simulink model "AM_07_model_pretvornik_FOC"  (R2016a)
settings: Solver=ode23  StartTime=0.0  StopTime=1  FixedStep=25e-9  MaxStep=1/(20*Fstikalna)  RelTol=1e-2
InitFcn:
  | parametriAM
values from neighbouring files (symbols this model uses):
  Imrn = 7.4    [parametriAM.m]
  In = 12.7    [parametriAM.m]
  Ismax = In*sqrt(2)    [parametriAM.m]
  J = 0.019    [parametriAM.m]    (also in podatki.m = 0.01)
  Ki_tok = 5.0    (= 5)    [parametriAM.m]
  Ki_wr = 1000    [parametriAM.m]
  Kp_tok = 0.05    [parametriAM.m]
  Kp_wr = 50    [parametriAM.m]
  Lm = 0.0493    [parametriAM.m]    (also in podatki.m = 0.2342)
  Lr = 0.05315    [parametriAM.m]    (also in podatki.m = 0.2449)
  Ls = 0.05315    [parametriAM.m]    (also in podatki.m = 0.2449)
  Lst = sigma*Ls    (= 0.00742111947319)    [parametriAM.m]
  pp = 3    [parametriAM.m]    (also in podatki.m = 2)
  sigma = 1 - 1/((1+sigmaR)*(1+sigmaS))    (= 0.13962595434)    [parametriAM.m]
  Tr = Lr/Rr    (= 0.0771407837446)    [parametriAM.m]
  Tstikalna = 1/Fstikalna    (= 0.0001)    [parametriAM.m]
  Udc = Un*sqrt(2/3*2)    [parametriAM.m]
  Un = 216    [parametriAM.m]
  wb_upper_limit_field_weaking = sqrt((Ls^2+Lst^2)/(2*Lst^2*Ls^2))*Un/Ismax    [parametriAM.m]
  wn = Udc/sqrt(Ls^2*(Imrn)^2+Lst^2*(Ismax^2-(Imrn)^2))    [maximalnaelipsa.m]    (also in parametriAM.m = Udc/sqrt(Ls^2*(Imrn)^2+Lst^2*(Ismax^2-(Imrn)^2))/pp/sqrt(2))
undefined symbols (not defined in the file or in its folder): DiscIntNeverNeededParam
undefined symbols (not defined in the file): Rr, Rs
libraries: simulink x23, simulink_extras x3
(part 2 of 2)

== system AM_07_model_pretvornik_FOC/Regulacija1/tokovni_model ==
  I_123 : Inport
  wr : Inport  Port=2
  Clarke : Subsystem
  Demux : Demux  Outputs=2
  Discrete-Time Integrator : DiscreteIntegrator  SampleTime=-1  ICPrevOutput=DiscIntNeverNeededParam  ICPrevScaledInput=DiscIntNeverNeededParam
  Gain : Gain  Gain=pp
  Park : Subsystem
  Terminator : Terminator
  eq 5.39 : Subsystem
  eq 5.40 : Subsystem
  I_dq : Outport
  Imr : Outport  Port=2
  ro : Outport  Port=3
  wires:
  wr/1 -> Gain/1
  eq 5.39/2(dImr/dt) -> Terminator/1
  Discrete-Time Integrator/1 -> Park/2(kot), ro/1
  eq 5.40/1(wmr) -> Discrete-Time Integrator/1
  Gain/1 -> eq 5.40/3(wr_el)
  Demux/2 -> eq 5.40/2(Isq)
  eq 5.39/1(Imr) -> Imr/1, eq 5.40/1(Imr)
  Demux/1 -> eq 5.39/1(Isd)
  I_123/1 -> Clarke/1(U_123)
  Clarke/1(U_ab) -> Park/1(U_ab)
  Park/1(U_dq) -> Demux/1, I_dq/1

== system AM_07_model_pretvornik_FOC/Regulacija2/Inverzni Park ==
  U_dq : Inport
  kot : Inport  Port=2
  Demux : Demux  Outputs=2
  Mux : Mux  Inputs=2
  "Sum1 " : Sum  Inputs=+-  SaturateOnIntegerOverflow=on  InputSameDT=on  OutDataTypeStr=Inherit: Same as first input
  Sum2 : Sum  SaturateOnIntegerOverflow=on  InputSameDT=on  OutDataTypeStr=Inherit: Same as first input
  cos : Fcn  Expr=cos(u)
  sin : Fcn  Expr=sin(u)
  x_d*cos : Product  SaturateOnIntegerOverflow=on  RndMeth=Zero  InputSameDT=on  OutDataTypeStr=Inherit: Same as first input
  x_d*sin : Product  SaturateOnIntegerOverflow=on  RndMeth=Zero  InputSameDT=on  OutDataTypeStr=Inherit: Same as first input
  x_q*cos : Product  SaturateOnIntegerOverflow=on  RndMeth=Zero  InputSameDT=on  OutDataTypeStr=Inherit: Same as first input
  "x_q*sin " : Product  SaturateOnIntegerOverflow=on  RndMeth=Zero  InputSameDT=on  OutDataTypeStr=Inherit: Same as first input
  U_ab : Outport
  wires:
  kot/1 -> sin/1, cos/1
  Sum2/1 -> Mux/2
  "Sum1 "/1 -> Mux/1
  x_d*sin/1 -> Sum2/1
  x_q*cos/1 -> Sum2/2
  "x_q*sin "/1 -> "Sum1 "/2
  x_d*cos/1 -> "Sum1 "/1
  sin/1 -> x_d*sin/2, "x_q*sin "/2
  cos/1 -> x_d*cos/2, x_q*cos/2
  Demux/2 -> x_q*cos/1, "x_q*sin "/1
  Demux/1 -> x_d*cos/1, x_d*sin/1
  U_dq/1 -> Demux/1
  Mux/1 -> U_ab/1

== system AM_07_model_pretvornik_FOC/Regulacija2/TechniqueA2 ==
  wmr : Inport
  Abs : Abs
  Add : Sum
  Constant : Constant  Value=wn
  Constant1 : Constant  Value=0.000001
  Constant2 : Constant  Value=Imrn
  Divide : Product  Inputs=*/
  Product : Product
  Saturation : Saturate  UpperLimit=+Imrn*sqrt(2)  LowerLimit=-Imrn*sqrt(2)
  Saturation2 : Saturate  UpperLimit=wb_upper_limit_field_weaking  LowerLimit=-wb_upper_limit_field_weaking
  Nemec : Outport
  wires:
  Saturation2/1 -> Abs/1
  Saturation/1 -> Nemec/1
  Constant1/1 -> Add/2
  Abs/1 -> Add/1
  Add/1 -> Divide/2
  Constant/1 -> Divide/1
  Product/1 -> Saturation/1
  Divide/1 -> Product/2
  Constant2/1 -> Product/1
  wmr/1 -> Saturation2/1

== system AM_07_model_pretvornik_FOC/Regulacija2/hitrostna regulacija ==
  ref : Inport
  fdb : Inport  Port=2
  1/Ti : Gain  Gain=Ki_wr  SaturateOnIntegerOverflow=on  OutDataTypeStr=Inherit: Same as input  ParamDataTypeStr=Inherit: Same as input
  Abs : Abs
  Add2 : Sum  Inputs=+-
  Compare To Zero : simulink/Logic and Bit Operations/Compare To Zero  relop=<=  OutDataTypeStr=boolean
  Discrete-Time Integrator : DiscreteIntegrator  SampleTime=-1  ICPrevOutput=DiscIntNeverNeededParam  ICPrevScaledInput=DiscIntNeverNeededParam
  Kp : Gain  Gain=Kp_wr  SaturateOnIntegerOverflow=on  OutDataTypeStr=Inherit: Same as input  ParamDataTypeStr=Inherit: Same as input
  Product : Product
  Saturation : Saturate  UpperLimit=+sqrt((In^2 - Imrn^2))*sqrt(2)  LowerLimit=-sqrt((In^2 - Imrn^2))*sqrt(2)
  Sum1 : Sum  Inputs=|+-
  Sum2 : Sum  Inputs=|++
  U_out : Outport
  wires:
  Saturation/1 -> Add2/2, U_out/1
  Kp/1 -> Sum2/1
  1/Ti/1 -> Discrete-Time Integrator/1
  Sum1/1 -> Product/1, Kp/1
  ref/1 -> Sum1/1
  fdb/1 -> Sum1/2
  Discrete-Time Integrator/1 -> Sum2/2
  Sum2/1 -> Add2/1, Saturation/1
  Add2/1 -> Abs/1
  Abs/1 -> Compare To Zero/1
  Compare To Zero/1 -> Product/2
  Product/1 -> 1/Ti/1

== system AM_07_model_pretvornik_FOC/Regulacija2/tokovna regulacija d ==
  ref : Inport
  fdb : Inport  Port=2
  1/Ti : Gain  Gain=Ki_tok  SaturateOnIntegerOverflow=on  OutDataTypeStr=Inherit: Same as input  ParamDataTypeStr=Inherit: Same as input
  Abs : Abs
  Add2 : Sum  Inputs=+-
  Compare To Zero : simulink/Logic and Bit Operations/Compare To Zero  relop=<=  OutDataTypeStr=boolean
  Discrete-Time Integrator : DiscreteIntegrator  SampleTime=-1  ICPrevOutput=DiscIntNeverNeededParam  ICPrevScaledInput=DiscIntNeverNeededParam
  Kp : Gain  Gain=Kp_tok  SaturateOnIntegerOverflow=on  OutDataTypeStr=Inherit: Same as input  ParamDataTypeStr=Inherit: Same as input
  Product : Product
  Saturation : Saturate  UpperLimit=+0.99  LowerLimit=-0.99
  Sum1 : Sum  Inputs=|+-
  Sum2 : Sum  Inputs=|++
  out : Outport
  wires:
  Saturation/1 -> Add2/2, out/1
  Kp/1 -> Sum2/1
  1/Ti/1 -> Discrete-Time Integrator/1
  Sum1/1 -> Product/1, Kp/1
  ref/1 -> Sum1/1
  fdb/1 -> Sum1/2
  Discrete-Time Integrator/1 -> Sum2/2
  Sum2/1 -> Add2/1, Saturation/1
  Add2/1 -> Abs/1
  Abs/1 -> Compare To Zero/1
  Compare To Zero/1 -> Product/2
  Product/1 -> 1/Ti/1

== system AM_07_model_pretvornik_FOC/Regulacija2/tokovna regulacija q ==
  ref : Inport
  fdb : Inport  Port=2
  1/Ti : Gain  Gain=Ki_tok  SaturateOnIntegerOverflow=on  OutDataTypeStr=Inherit: Same as input  ParamDataTypeStr=Inherit: Same as input
  Abs : Abs
  Add2 : Sum  Inputs=+-
  Compare To Zero : simulink/Logic and Bit Operations/Compare To Zero  relop=<=  OutDataTypeStr=boolean
  Discrete-Time Integrator : DiscreteIntegrator  SampleTime=-1  ICPrevOutput=DiscIntNeverNeededParam  ICPrevScaledInput=DiscIntNeverNeededParam
  Kp : Gain  Gain=Kp_tok  SaturateOnIntegerOverflow=on  OutDataTypeStr=Inherit: Same as input  ParamDataTypeStr=Inherit: Same as input
  Product : Product
  Saturation : Saturate  UpperLimit=+0.99  LowerLimit=-0.99
  Sum1 : Sum  Inputs=|+-
  Sum2 : Sum  Inputs=|++
  out : Outport
  wires:
  Saturation/1 -> Add2/2, out/1
  Kp/1 -> Sum2/1
  1/Ti/1 -> Discrete-Time Integrator/1
  Sum1/1 -> Product/1, Kp/1
  ref/1 -> Sum1/1
  fdb/1 -> Sum1/2
  Discrete-Time Integrator/1 -> Sum2/2
  Sum2/1 -> Add2/1, Saturation/1
  Add2/1 -> Abs/1
  Abs/1 -> Compare To Zero/1
  Compare To Zero/1 -> Product/2
  Product/1 -> 1/Ti/1

== system AM_07_model_pretvornik_FOC/Regulacija2/tokovni_model ==
  I_123 : Inport
  wr : Inport  Port=2
  Clarke : Subsystem
  Demux : Demux  Outputs=2
  Discrete-Time Integrator : DiscreteIntegrator  SampleTime=-1  ICPrevOutput=DiscIntNeverNeededParam  ICPrevScaledInput=DiscIntNeverNeededParam
  Gain : Gain  Gain=pp
  Park : Subsystem
  Terminator : Terminator
  eq 5.39 : Subsystem
  eq 5.40 : Subsystem
  I_dq : Outport
  Imr : Outport  Port=2
  ro : Outport  Port=3
  wires:
  Park/1(U_dq) -> I_dq/1, Demux/1
  Clarke/1(U_ab) -> Park/1(U_ab)
  I_123/1 -> Clarke/1(U_123)
  Demux/1 -> eq 5.39/1(Isd)
  eq 5.39/1(Imr) -> eq 5.40/1(Imr), Imr/1
  Demux/2 -> eq 5.40/2(Isq)
  Gain/1 -> eq 5.40/3(wr_el)
  eq 5.40/1(wmr) -> Discrete-Time Integrator/1
  Discrete-Time Integrator/1 -> ro/1, Park/2(kot)
  eq 5.39/2(dImr/dt) -> Terminator/1
  wr/1 -> Gain/1

== system AM_07_model_pretvornik_FOC/ACIM_model/Elektricni del1/Clarke ==
  U_123 : Inport
  ABC_ab1 : Subsystem
  Demux : Demux  Outputs=3
  Mux : Mux  Inputs=2
  U_ab : Outport
  wires:
  U_123/1 -> Demux/1
  Demux/1 -> ABC_ab1/1(A)
  Demux/2 -> ABC_ab1/2(B)
  Demux/3 -> ABC_ab1/3(C)
  ABC_ab1/1(alfa) -> Mux/1
  ABC_ab1/2(beta) -> Mux/2
  Mux/1 -> U_ab/1

== system AM_07_model_pretvornik_FOC/ACIM_model/Elektricni del1/Inverzni Clarke ==
  I_ab : Inport
  Demux : Demux  Outputs=2
  Mux : Mux  Inputs=3
  ab_ABC : Subsystem
  I_123 : Outport
  wires:
  Mux/1 -> I_123/1
  I_ab/1 -> Demux/1
  Demux/1 -> ab_ABC/1(alfa)
  Demux/2 -> ab_ABC/2(beta)
  ab_ABC/1(A) -> Mux/1
  ab_ABC/2(B) -> Mux/2
  ab_ABC/3(C) -> Mux/3

== system AM_07_model_pretvornik_FOC/ACIM_model/Elektricni del1/Inverzni Park ==
  I_dq : Inport
  kot : Inport  Port=2
  Demux : Demux  Outputs=2
  Mux : Mux  Inputs=2
  "Sum1 " : Sum  Inputs=+-  SaturateOnIntegerOverflow=on  InputSameDT=on  OutDataTypeStr=Inherit: Same as first input
  Sum2 : Sum  SaturateOnIntegerOverflow=on  InputSameDT=on  OutDataTypeStr=Inherit: Same as first input
  cos : Fcn  Expr=cos(u)
  sin : Fcn  Expr=sin(u)
  x_d*cos : Product  SaturateOnIntegerOverflow=on  RndMeth=Zero  InputSameDT=on  OutDataTypeStr=Inherit: Same as first input
  x_d*sin : Product  SaturateOnIntegerOverflow=on  RndMeth=Zero  InputSameDT=on  OutDataTypeStr=Inherit: Same as first input
  x_q*cos : Product  SaturateOnIntegerOverflow=on  RndMeth=Zero  InputSameDT=on  OutDataTypeStr=Inherit: Same as first input
  "x_q*sin " : Product  SaturateOnIntegerOverflow=on  RndMeth=Zero  InputSameDT=on  OutDataTypeStr=Inherit: Same as first input
  I_ab : Outport
  wires:
  kot/1 -> sin/1, cos/1
  Sum2/1 -> Mux/2
  "Sum1 "/1 -> Mux/1
  x_d*sin/1 -> Sum2/1
  x_q*cos/1 -> Sum2/2
  "x_q*sin "/1 -> "Sum1 "/2
  x_d*cos/1 -> "Sum1 "/1
  sin/1 -> x_d*sin/2, "x_q*sin "/2
  cos/1 -> x_d*cos/2, x_q*cos/2
  Demux/2 -> x_q*cos/1, "x_q*sin "/1
  Demux/1 -> x_d*cos/1, x_d*sin/1
  I_dq/1 -> Demux/1
  Mux/1 -> I_ab/1

== system AM_07_model_pretvornik_FOC/ACIM_model/Elektricni del1/Park ==
  U_ab : Inport
  kot : Inport  Port=2
  Demux : Demux  Outputs=2
  Mux : Mux  Inputs=2
  "Sum1 " : Sum  SaturateOnIntegerOverflow=on  InputSameDT=on  OutDataTypeStr=Inherit: Same as first input
  Sum2 : Sum  Inputs=-+  SaturateOnIntegerOverflow=on  InputSameDT=on  OutDataTypeStr=Inherit: Same as first input
  cos : Fcn  Expr=cos(u)
  sin : Fcn  Expr=sin(u)
  x_a*cos : Product  SaturateOnIntegerOverflow=on  RndMeth=Zero  InputSameDT=on  OutDataTypeStr=Inherit: Same as first input
  x_a*sin : Product  SaturateOnIntegerOverflow=on  RndMeth=Zero  InputSameDT=on  OutDataTypeStr=Inherit: Same as first input
  x_b*cos : Product  SaturateOnIntegerOverflow=on  RndMeth=Zero  InputSameDT=on  OutDataTypeStr=Inherit: Same as first input
  "x_b*sin " : Product  SaturateOnIntegerOverflow=on  RndMeth=Zero  InputSameDT=on  OutDataTypeStr=Inherit: Same as first input
  U_dq : Outport
  wires:
  kot/1 -> sin/1, cos/1
  Sum2/1 -> Mux/2
  "Sum1 "/1 -> Mux/1
  x_a*sin/1 -> Sum2/1
  x_b*cos/1 -> Sum2/2
  "x_b*sin "/1 -> "Sum1 "/2
  x_a*cos/1 -> "Sum1 "/1
  sin/1 -> x_a*sin/2, "x_b*sin "/2
  cos/1 -> x_a*cos/2, x_b*cos/2
  Demux/2 -> x_b*cos/1, "x_b*sin "/1
  Demux/1 -> x_a*cos/1, x_a*sin/1
  U_ab/1 -> Demux/1
  Mux/1 -> U_dq/1

== system AM_07_model_pretvornik_FOC/ACIM_model/Elektricni del1/napetostni dq model ==
  Us_dq : Inport
  wr : Inport  Port=2
  Demux : Demux  Outputs=2
  Gain : Gain  Gain=pp
  Integrator : Integrator
  Mux : Mux  Inputs=2
  eq 5.35 : Subsystem
  eq 5.39 : Subsystem
  eq 5.40 : Subsystem
  eq 5.46 : Subsystem
  eq 5.47 : Subsystem
  Mel : Outport
  Is_dq : Outport  Port=2
  ro : Outport  Port=3
  wires:
  eq 5.46/1(Isd) -> eq 5.39/1(Isd), eq 5.47/3(Isd), Mux/1
  eq 5.39/2(dImr/dt) -> eq 5.46/2(dImr/dt)
  eq 5.39/1(Imr) -> eq 5.35/1(Imr), eq 5.40/1(Imr), eq 5.47/2(Imr)
  eq 5.47/1(Isq) -> eq 5.35/2(Isq), eq 5.40/2(Isq), eq 5.46/3(Isq), Mux/2
  eq 5.40/1(w_mr) -> eq 5.47/4(wmr), eq 5.46/4(wmr), Integrator/1
  eq 5.35/1(Mel) -> Mel/1
  Integrator/1 -> ro/1
  wr/1 -> Gain/1
  Us_dq/1 -> Demux/1
  Demux/1 -> eq 5.46/1(Usd)
  Demux/2 -> eq 5.47/1(Usq)
  Mux/1 -> Is_dq/1
  Gain/1 -> eq 5.40/3(wr_el)

== system AM_07_model_pretvornik_FOC/ACIM_model/Mehanika/eq 2.19 ==
  M : Inport
  Gain1 : Gain  Gain=1/J
  Integrator : Integrator
  wr : Outport
  wires:
  Gain1/1 -> Integrator/1
  M/1 -> Gain1/1
  Integrator/1 -> wr/1

== system AM_07_model_pretvornik_FOC/ACIM_model/Mehanika/trenje in zracni upor ==
  wr : Inport
  Gain2 : Gain  Gain=Ktrenja
  Gain3 : Gain  Gain=Kupora
  Rate Limiter : RateLimiter  RisingSlewLimit=10000  FallingSlewLimit=-10000  SampleTimeMode=inherited
  Sign : Signum  ZeroCross=off
  Sum : Sum  Inputs=|++
  Mtrenja : Outport
  wires:
  wr/1 -> Gain3/1, Sign/1
  Sum/1 -> Mtrenja/1
  Gain2/1 -> Sum/1
  Gain3/1 -> Sum/2
  Sign/1 -> Rate Limiter/1
  Rate Limiter/1 -> Gain2/1

== system AM_07_model_pretvornik_FOC/ACIM_model1/Elektricni del1/Clarke ==
  U_123 : Inport
  ABC_ab1 : Subsystem
  Demux : Demux  Outputs=3
  Mux : Mux  Inputs=2
  U_ab : Outport
  wires:
  Mux/1 -> U_ab/1
  ABC_ab1/2(beta) -> Mux/2
  ABC_ab1/1(alfa) -> Mux/1
  Demux/3 -> ABC_ab1/3(C)
  Demux/2 -> ABC_ab1/2(B)
  Demux/1 -> ABC_ab1/1(A)
  U_123/1 -> Demux/1

== system AM_07_model_pretvornik_FOC/ACIM_model1/Elektricni del1/Inverzni Clarke ==
  I_ab : Inport
  Demux : Demux  Outputs=2
  Mux : Mux  Inputs=3
  ab_ABC : Subsystem
  I_123 : Outport
  wires:
  ab_ABC/3(C) -> Mux/3
  ab_ABC/2(B) -> Mux/2
  ab_ABC/1(A) -> Mux/1
  Demux/2 -> ab_ABC/2(beta)
  Demux/1 -> ab_ABC/1(alfa)
  I_ab/1 -> Demux/1
  Mux/1 -> I_123/1

== system AM_07_model_pretvornik_FOC/ACIM_model1/Elektricni del1/Inverzni Park ==
  I_dq : Inport
  kot : Inport  Port=2
  Demux : Demux  Outputs=2
  Mux : Mux  Inputs=2
  "Sum1 " : Sum  Inputs=+-  SaturateOnIntegerOverflow=on  InputSameDT=on  OutDataTypeStr=Inherit: Same as first input
  Sum2 : Sum  SaturateOnIntegerOverflow=on  InputSameDT=on  OutDataTypeStr=Inherit: Same as first input
  cos : Fcn  Expr=cos(u)
  sin : Fcn  Expr=sin(u)
  x_d*cos : Product  SaturateOnIntegerOverflow=on  RndMeth=Zero  InputSameDT=on  OutDataTypeStr=Inherit: Same as first input
  x_d*sin : Product  SaturateOnIntegerOverflow=on  RndMeth=Zero  InputSameDT=on  OutDataTypeStr=Inherit: Same as first input
  x_q*cos : Product  SaturateOnIntegerOverflow=on  RndMeth=Zero  InputSameDT=on  OutDataTypeStr=Inherit: Same as first input
  "x_q*sin " : Product  SaturateOnIntegerOverflow=on  RndMeth=Zero  InputSameDT=on  OutDataTypeStr=Inherit: Same as first input
  I_ab : Outport
  wires:
  Mux/1 -> I_ab/1
  I_dq/1 -> Demux/1
  Demux/1 -> x_d*sin/1, x_d*cos/1
  Demux/2 -> "x_q*sin "/1, x_q*cos/1
  cos/1 -> x_q*cos/2, x_d*cos/2
  sin/1 -> "x_q*sin "/2, x_d*sin/2
  x_d*cos/1 -> "Sum1 "/1
  "x_q*sin "/1 -> "Sum1 "/2
  x_q*cos/1 -> Sum2/2
  x_d*sin/1 -> Sum2/1
  "Sum1 "/1 -> Mux/1
  Sum2/1 -> Mux/2
  kot/1 -> cos/1, sin/1

== system AM_07_model_pretvornik_FOC/ACIM_model1/Elektricni del1/Park ==
  U_ab : Inport
  kot : Inport  Port=2
  Demux : Demux  Outputs=2
  Mux : Mux  Inputs=2
  "Sum1 " : Sum  SaturateOnIntegerOverflow=on  InputSameDT=on  OutDataTypeStr=Inherit: Same as first input
  Sum2 : Sum  Inputs=-+  SaturateOnIntegerOverflow=on  InputSameDT=on  OutDataTypeStr=Inherit: Same as first input
  cos : Fcn  Expr=cos(u)
  sin : Fcn  Expr=sin(u)
  x_a*cos : Product  SaturateOnIntegerOverflow=on  RndMeth=Zero  InputSameDT=on  OutDataTypeStr=Inherit: Same as first input
  x_a*sin : Product  SaturateOnIntegerOverflow=on  RndMeth=Zero  InputSameDT=on  OutDataTypeStr=Inherit: Same as first input
  x_b*cos : Product  SaturateOnIntegerOverflow=on  RndMeth=Zero  InputSameDT=on  OutDataTypeStr=Inherit: Same as first input
  "x_b*sin " : Product  SaturateOnIntegerOverflow=on  RndMeth=Zero  InputSameDT=on  OutDataTypeStr=Inherit: Same as first input
  U_dq : Outport
  wires:
  Mux/1 -> U_dq/1
  U_ab/1 -> Demux/1
  Demux/1 -> x_a*sin/1, x_a*cos/1
  Demux/2 -> "x_b*sin "/1, x_b*cos/1
  cos/1 -> x_b*cos/2, x_a*cos/2
  sin/1 -> "x_b*sin "/2, x_a*sin/2
  x_a*cos/1 -> "Sum1 "/1
  "x_b*sin "/1 -> "Sum1 "/2
  x_b*cos/1 -> Sum2/2
  x_a*sin/1 -> Sum2/1
  "Sum1 "/1 -> Mux/1
  Sum2/1 -> Mux/2
  kot/1 -> cos/1, sin/1

== system AM_07_model_pretvornik_FOC/ACIM_model1/Elektricni del1/napetostni dq model ==
  Us_dq : Inport
  wr : Inport  Port=2
  Demux : Demux  Outputs=2
  Gain : Gain  Gain=pp
  Integrator : Integrator
  Mux : Mux  Inputs=2
  eq 5.35 : Subsystem
  eq 5.39 : Subsystem
  eq 5.40 : Subsystem
  eq 5.46 : Subsystem
  eq 5.47 : Subsystem
  Mel : Outport
  Is_dq : Outport  Port=2
  ro : Outport  Port=3
  wires:
  Gain/1 -> eq 5.40/3(wr_el)
  Mux/1 -> Is_dq/1
  Demux/2 -> eq 5.47/1(Usq)
  Demux/1 -> eq 5.46/1(Usd)
  Us_dq/1 -> Demux/1
  wr/1 -> Gain/1
  Integrator/1 -> ro/1
  eq 5.35/1(Mel) -> Mel/1
  eq 5.40/1(w_mr) -> Integrator/1, eq 5.46/4(wmr), eq 5.47/4(wmr)
  eq 5.47/1(Isq) -> Mux/2, eq 5.46/3(Isq), eq 5.40/2(Isq), eq 5.35/2(Isq)
  eq 5.39/1(Imr) -> eq 5.47/2(Imr), eq 5.40/1(Imr), eq 5.35/1(Imr)
  eq 5.39/2(dImr/dt) -> eq 5.46/2(dImr/dt)
  eq 5.46/1(Isd) -> Mux/1, eq 5.47/3(Isd), eq 5.39/1(Isd)

== system AM_07_model_pretvornik_FOC/ACIM_model1/Mehanika/eq 2.19 ==
  M : Inport
  Gain1 : Gain  Gain=1/J
  Integrator : Integrator
  wr : Outport
  wires:
  Integrator/1 -> wr/1
  M/1 -> Gain1/1
  Gain1/1 -> Integrator/1

== system AM_07_model_pretvornik_FOC/ACIM_model1/Mehanika/trenje in zracni upor ==
  wr : Inport
  Gain2 : Gain  Gain=Ktrenja
  Gain3 : Gain  Gain=Kupora
  Rate Limiter : RateLimiter  RisingSlewLimit=10000  FallingSlewLimit=-10000  SampleTimeMode=inherited
  Sign : Signum  ZeroCross=off
  Sum : Sum  Inputs=|++
  Mtrenja : Outport
  wires:
  Rate Limiter/1 -> Gain2/1
  Sign/1 -> Rate Limiter/1
  Gain3/1 -> Sum/2
  Gain2/1 -> Sum/1
  Sum/1 -> Mtrenja/1
  wr/1 -> Sign/1, Gain3/1

== system AM_07_model_pretvornik_FOC/ACIM_model2/Elektricni del1/Clarke ==
  U_123 : Inport
  ABC_ab1 : Subsystem
  Demux : Demux  Outputs=3
  Mux : Mux  Inputs=2
  U_ab : Outport
  wires:
  U_123/1 -> Demux/1
  Demux/1 -> ABC_ab1/1(A)
  Demux/2 -> ABC_ab1/2(B)
  Demux/3 -> ABC_ab1/3(C)
  ABC_ab1/1(alfa) -> Mux/1
  ABC_ab1/2(beta) -> Mux/2
  Mux/1 -> U_ab/1

== system AM_07_model_pretvornik_FOC/ACIM_model2/Elektricni del1/Inverzni Clarke ==
  I_ab : Inport
  Demux : Demux  Outputs=2
  Mux : Mux  Inputs=3
  ab_ABC : Subsystem
  I_123 : Outport
  wires:
  Mux/1 -> I_123/1
  I_ab/1 -> Demux/1
  Demux/1 -> ab_ABC/1(alfa)
  Demux/2 -> ab_ABC/2(beta)
  ab_ABC/1(A) -> Mux/1
  ab_ABC/2(B) -> Mux/2
  ab_ABC/3(C) -> Mux/3

== system AM_07_model_pretvornik_FOC/ACIM_model2/Elektricni del1/Inverzni Park ==
  I_dq : Inport
  kot : Inport  Port=2
  Demux : Demux  Outputs=2
  Mux : Mux  Inputs=2
  "Sum1 " : Sum  Inputs=+-  SaturateOnIntegerOverflow=on  InputSameDT=on  OutDataTypeStr=Inherit: Same as first input
  Sum2 : Sum  SaturateOnIntegerOverflow=on  InputSameDT=on  OutDataTypeStr=Inherit: Same as first input
  cos : Fcn  Expr=cos(u)
  sin : Fcn  Expr=sin(u)
  x_d*cos : Product  SaturateOnIntegerOverflow=on  RndMeth=Zero  InputSameDT=on  OutDataTypeStr=Inherit: Same as first input
  x_d*sin : Product  SaturateOnIntegerOverflow=on  RndMeth=Zero  InputSameDT=on  OutDataTypeStr=Inherit: Same as first input
  x_q*cos : Product  SaturateOnIntegerOverflow=on  RndMeth=Zero  InputSameDT=on  OutDataTypeStr=Inherit: Same as first input
  "x_q*sin " : Product  SaturateOnIntegerOverflow=on  RndMeth=Zero  InputSameDT=on  OutDataTypeStr=Inherit: Same as first input
  I_ab : Outport
  wires:
  kot/1 -> sin/1, cos/1
  Sum2/1 -> Mux/2
  "Sum1 "/1 -> Mux/1
  x_d*sin/1 -> Sum2/1
  x_q*cos/1 -> Sum2/2
  "x_q*sin "/1 -> "Sum1 "/2
  x_d*cos/1 -> "Sum1 "/1
  sin/1 -> x_d*sin/2, "x_q*sin "/2
  cos/1 -> x_d*cos/2, x_q*cos/2
  Demux/2 -> x_q*cos/1, "x_q*sin "/1
  Demux/1 -> x_d*cos/1, x_d*sin/1
  I_dq/1 -> Demux/1
  Mux/1 -> I_ab/1

== system AM_07_model_pretvornik_FOC/ACIM_model2/Elektricni del1/Park ==
  U_ab : Inport
  kot : Inport  Port=2
  Demux : Demux  Outputs=2
  Mux : Mux  Inputs=2
  "Sum1 " : Sum  SaturateOnIntegerOverflow=on  InputSameDT=on  OutDataTypeStr=Inherit: Same as first input
  Sum2 : Sum  Inputs=-+  SaturateOnIntegerOverflow=on  InputSameDT=on  OutDataTypeStr=Inherit: Same as first input
  cos : Fcn  Expr=cos(u)
  sin : Fcn  Expr=sin(u)
  x_a*cos : Product  SaturateOnIntegerOverflow=on  RndMeth=Zero  InputSameDT=on  OutDataTypeStr=Inherit: Same as first input
  x_a*sin : Product  SaturateOnIntegerOverflow=on  RndMeth=Zero  InputSameDT=on  OutDataTypeStr=Inherit: Same as first input
  x_b*cos : Product  SaturateOnIntegerOverflow=on  RndMeth=Zero  InputSameDT=on  OutDataTypeStr=Inherit: Same as first input
  "x_b*sin " : Product  SaturateOnIntegerOverflow=on  RndMeth=Zero  InputSameDT=on  OutDataTypeStr=Inherit: Same as first input
  U_dq : Outport
  wires:
  kot/1 -> sin/1, cos/1
  Sum2/1 -> Mux/2
  "Sum1 "/1 -> Mux/1
  x_a*sin/1 -> Sum2/1
  x_b*cos/1 -> Sum2/2
  "x_b*sin "/1 -> "Sum1 "/2
  x_a*cos/1 -> "Sum1 "/1
  sin/1 -> x_a*sin/2, "x_b*sin "/2
  cos/1 -> x_a*cos/2, x_b*cos/2
  Demux/2 -> x_b*cos/1, "x_b*sin "/1
  Demux/1 -> x_a*cos/1, x_a*sin/1
  U_ab/1 -> Demux/1
  Mux/1 -> U_dq/1

== system AM_07_model_pretvornik_FOC/ACIM_model2/Elektricni del1/napetostni dq model ==
  Us_dq : Inport
  wr : Inport  Port=2
  Demux : Demux  Outputs=2
  Gain : Gain  Gain=pp
  Integrator : Integrator
  Mux : Mux  Inputs=2
  eq 5.35 : Subsystem
  eq 5.39 : Subsystem
  eq 5.40 : Subsystem
  eq 5.46 : Subsystem
  eq 5.47 : Subsystem
  Mel : Outport
  Is_dq : Outport  Port=2
  ro : Outport  Port=3
  wires:
  eq 5.46/1(Isd) -> eq 5.39/1(Isd), eq 5.47/3(Isd), Mux/1
  eq 5.39/2(dImr/dt) -> eq 5.46/2(dImr/dt)
  eq 5.39/1(Imr) -> eq 5.35/1(Imr), eq 5.40/1(Imr), eq 5.47/2(Imr)
  eq 5.47/1(Isq) -> eq 5.35/2(Isq), eq 5.40/2(Isq), eq 5.46/3(Isq), Mux/2
  eq 5.40/1(w_mr) -> eq 5.47/4(wmr), eq 5.46/4(wmr), Integrator/1
  eq 5.35/1(Mel) -> Mel/1
  Integrator/1 -> ro/1
  wr/1 -> Gain/1
  Us_dq/1 -> Demux/1
  Demux/1 -> eq 5.46/1(Usd)
  Demux/2 -> eq 5.47/1(Usq)
  Mux/1 -> Is_dq/1
  Gain/1 -> eq 5.40/3(wr_el)

== system AM_07_model_pretvornik_FOC/ACIM_model2/Mehanika/eq 2.19 ==
  M : Inport
  Gain1 : Gain  Gain=1/J
  Integrator : Integrator
  wr : Outport
  wires:
  Gain1/1 -> Integrator/1
  M/1 -> Gain1/1
  Integrator/1 -> wr/1

== system AM_07_model_pretvornik_FOC/ACIM_model2/Mehanika/trenje in zracni upor ==
  wr : Inport
  Gain2 : Gain  Gain=Ktrenja
  Gain3 : Gain  Gain=Kupora
  Rate Limiter : RateLimiter  RisingSlewLimit=10000  FallingSlewLimit=-10000  SampleTimeMode=inherited
  Sign : Signum  ZeroCross=off
  Sum : Sum  Inputs=|++
  Mtrenja : Outport
  wires:
  wr/1 -> Gain3/1, Sign/1
  Sum/1 -> Mtrenja/1
  Gain2/1 -> Sum/1
  Gain3/1 -> Sum/2
  Sign/1 -> Rate Limiter/1
  Rate Limiter/1 -> Gain2/1

== system AM_07_model_pretvornik_FOC/Regulacija/tokovni_model/Clarke ==
  U_123 : Inport
  ABC_ab1 : Subsystem
  Demux : Demux  Outputs=3
  Mux : Mux  Inputs=2
  U_ab : Outport
  wires:
  U_123/1 -> Demux/1
  Demux/1 -> ABC_ab1/1(A)
  Demux/2 -> ABC_ab1/2(B)
  Demux/3 -> ABC_ab1/3(C)
  ABC_ab1/1(alfa) -> Mux/1
  ABC_ab1/2(beta) -> Mux/2
  Mux/1 -> U_ab/1

== system AM_07_model_pretvornik_FOC/Regulacija/tokovni_model/Park ==
  U_ab : Inport
  kot : Inport  Port=2
  Demux : Demux  Outputs=2
  Mux : Mux  Inputs=2
  "Sum1 " : Sum  SaturateOnIntegerOverflow=on  InputSameDT=on  OutDataTypeStr=Inherit: Same as first input
  Sum2 : Sum  Inputs=-+  SaturateOnIntegerOverflow=on  InputSameDT=on  OutDataTypeStr=Inherit: Same as first input
  cos : Fcn  Expr=cos(u)
  sin : Fcn  Expr=sin(u)
  x_a*cos : Product  SaturateOnIntegerOverflow=on  RndMeth=Zero  InputSameDT=on  OutDataTypeStr=Inherit: Same as first input
  x_a*sin : Product  SaturateOnIntegerOverflow=on  RndMeth=Zero  InputSameDT=on  OutDataTypeStr=Inherit: Same as first input
  x_b*cos : Product  SaturateOnIntegerOverflow=on  RndMeth=Zero  InputSameDT=on  OutDataTypeStr=Inherit: Same as first input
  "x_b*sin " : Product  SaturateOnIntegerOverflow=on  RndMeth=Zero  InputSameDT=on  OutDataTypeStr=Inherit: Same as first input
  U_dq : Outport
  wires:
  kot/1 -> sin/1, cos/1
  Sum2/1 -> Mux/2
  "Sum1 "/1 -> Mux/1
  x_a*sin/1 -> Sum2/1
  x_b*cos/1 -> Sum2/2
  "x_b*sin "/1 -> "Sum1 "/2
  x_a*cos/1 -> "Sum1 "/1
  sin/1 -> x_a*sin/2, "x_b*sin "/2
  cos/1 -> x_a*cos/2, x_b*cos/2
  Demux/2 -> x_b*cos/1, "x_b*sin "/1
  Demux/1 -> x_a*cos/1, x_a*sin/1
  U_ab/1 -> Demux/1
  Mux/1 -> U_dq/1

== system AM_07_model_pretvornik_FOC/Regulacija/tokovni_model/eq 5.39 ==
  Isd : Inport
  Discrete-Time Integrator : DiscreteIntegrator  SampleTime=-1  ICPrevOutput=DiscIntNeverNeededParam  ICPrevScaledInput=DiscIntNeverNeededParam
  Gain : Gain  Gain=1/Tr
  Sum : Sum  Inputs=|+-
  Imr : Outport
  dImr/dt : Outport  Port=2
  wires:
  Isd/1 -> Sum/1
  Discrete-Time Integrator/1 -> Imr/1, Sum/2
  Sum/1 -> Gain/1
  Gain/1 -> Discrete-Time Integrator/1, dImr/dt/1

== system AM_07_model_pretvornik_FOC/Regulacija/tokovni_model/eq 5.40 ==
  Imr : Inport
  Isq : Inport  Port=2
  wr_el : Inport  Port=3
  Add : Sum
  Constant : Constant  Value=0.0001
  Divide : Product  Inputs=*/
  Gain2 : Gain  Gain=Tr
  Sum : Sum  Inputs=|++
  wmr : Outport
  wires:
  Isq/1 -> Divide/1
  Imr/1 -> Gain2/1
  Divide/1 -> Sum/1
  wr_el/1 -> Sum/2
  Sum/1 -> wmr/1
  Gain2/1 -> Add/1
  Add/1 -> Divide/2
  Constant/1 -> Add/2

== system AM_07_model_pretvornik_FOC/Regulacija1/TechniqueB1/Const c ==
  Id : Inport
  Imr : Inport  Port=2
  Discrete-Time Integrator : DiscreteIntegrator  SampleTime=-1  ICPrevOutput=DiscIntNeverNeededParam  ICPrevScaledInput=DiscIntNeverNeededParam
  Gain1 : Gain  Gain=Lm^2/Lr
  Gain4 : Gain  Gain=1/1
  Sum1 : Sum  Inputs=|+-
  Sum2 : Sum  Inputs=|+-
  c : Outport
  wires:
  Discrete-Time Integrator/1 -> Sum2/2, c/1
  Gain4/1 -> Discrete-Time Integrator/1
  Sum2/1 -> Gain4/1
  Gain1/1 -> Sum2/1
  Sum1/1 -> Gain1/1
  Imr/1 -> Sum1/1
  Id/1 -> Sum1/2

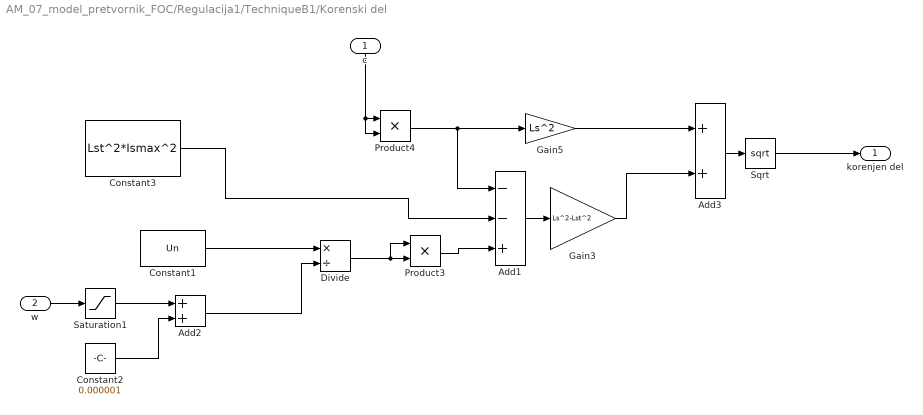
== system AM_07_model_pretvornik_FOC/Regulacija1/TechniqueB1/Korenski del ==
  c : Inport
  w : Inport  Port=2
  Add1 : Sum  Inputs=--+
  Add2 : Sum
  Add3 : Sum
  Constant1 : Constant  Value=Un
  Constant2 : Constant  Value=0.000001
  Constant3 : Constant  Value=Lst^2*Ismax^2
  Divide : Product  Inputs=*/
  Gain3 : Gain  Gain=Ls^2-Lst^2
  Gain5 : Gain  Gain=Ls^2
  Product3 : Product
  Product4 : Product
  Saturation1 : Saturate  UpperLimit=wb_upper_limit_field_weaking  LowerLimit=-wb_upper_limit_field_weaking
  Sqrt : Sqrt  SaturateOnIntegerOverflow=on
  korenjen del : Outport
  wires:
  c/1 -> Product4/2, Product4/1
  Product4/1 -> Add1/1, Gain5/1
  Saturation1/1 -> Add2/1
  Constant1/1 -> Divide/1
  Constant2/1 -> Add2/2
  Add1/1 -> Gain3/1
  Add2/1 -> Divide/2
  w/1 -> Saturation1/1
  Divide/1 -> Product3/1, Product3/2
  Product3/1 -> Add1/3
  Sqrt/1 -> korenjen del/1
  Add3/1 -> Sqrt/1
  Gain5/1 -> Add3/1
  Gain3/1 -> Add3/2
  Constant3/1 -> Add1/2

== system AM_07_model_pretvornik_FOC/Regulacija1/tokovni_model/Clarke ==
  U_123 : Inport
  ABC_ab1 : Subsystem
  Demux : Demux  Outputs=3
  Mux : Mux  Inputs=2
  U_ab : Outport
  wires:
  Mux/1 -> U_ab/1
  ABC_ab1/2(beta) -> Mux/2
  ABC_ab1/1(alfa) -> Mux/1
  Demux/3 -> ABC_ab1/3(C)
  Demux/2 -> ABC_ab1/2(B)
  Demux/1 -> ABC_ab1/1(A)
  U_123/1 -> Demux/1

== system AM_07_model_pretvornik_FOC/Regulacija1/tokovni_model/Park ==
  U_ab : Inport
  kot : Inport  Port=2
  Demux : Demux  Outputs=2
  Mux : Mux  Inputs=2
  "Sum1 " : Sum  SaturateOnIntegerOverflow=on  InputSameDT=on  OutDataTypeStr=Inherit: Same as first input
  Sum2 : Sum  Inputs=-+  SaturateOnIntegerOverflow=on  InputSameDT=on  OutDataTypeStr=Inherit: Same as first input
  cos : Fcn  Expr=cos(u)
  sin : Fcn  Expr=sin(u)
  x_a*cos : Product  SaturateOnIntegerOverflow=on  RndMeth=Zero  InputSameDT=on  OutDataTypeStr=Inherit: Same as first input
  x_a*sin : Product  SaturateOnIntegerOverflow=on  RndMeth=Zero  InputSameDT=on  OutDataTypeStr=Inherit: Same as first input
  x_b*cos : Product  SaturateOnIntegerOverflow=on  RndMeth=Zero  InputSameDT=on  OutDataTypeStr=Inherit: Same as first input
  "x_b*sin " : Product  SaturateOnIntegerOverflow=on  RndMeth=Zero  InputSameDT=on  OutDataTypeStr=Inherit: Same as first input
  U_dq : Outport
  wires:
  Mux/1 -> U_dq/1
  U_ab/1 -> Demux/1
  Demux/1 -> x_a*sin/1, x_a*cos/1
  Demux/2 -> "x_b*sin "/1, x_b*cos/1
  cos/1 -> x_b*cos/2, x_a*cos/2
  sin/1 -> "x_b*sin "/2, x_a*sin/2
  x_a*cos/1 -> "Sum1 "/1
  "x_b*sin "/1 -> "Sum1 "/2
  x_b*cos/1 -> Sum2/2
  x_a*sin/1 -> Sum2/1
  "Sum1 "/1 -> Mux/1
  Sum2/1 -> Mux/2
  kot/1 -> cos/1, sin/1

== system AM_07_model_pretvornik_FOC/Regulacija1/tokovni_model/eq 5.39 ==
  Isd : Inport
  Discrete-Time Integrator : DiscreteIntegrator  SampleTime=-1  ICPrevOutput=DiscIntNeverNeededParam  ICPrevScaledInput=DiscIntNeverNeededParam
  Gain : Gain  Gain=1/Tr
  Sum : Sum  Inputs=|+-
  Imr : Outport
  dImr/dt : Outport  Port=2
  wires:
  Gain/1 -> dImr/dt/1, Discrete-Time Integrator/1
  Sum/1 -> Gain/1
  Discrete-Time Integrator/1 -> Sum/2, Imr/1
  Isd/1 -> Sum/1

== system AM_07_model_pretvornik_FOC/Regulacija1/tokovni_model/eq 5.40 ==
  Imr : Inport
  Isq : Inport  Port=2
  wr_el : Inport  Port=3
  Add : Sum
  Constant : Constant  Value=0.0001
  Divide : Product  Inputs=*/
  Gain2 : Gain  Gain=Tr
  Sum : Sum  Inputs=|++
  wmr : Outport
  wires:
  Constant/1 -> Add/2
  Add/1 -> Divide/2
  Gain2/1 -> Add/1
  Sum/1 -> wmr/1
  wr_el/1 -> Sum/2
  Divide/1 -> Sum/1
  Imr/1 -> Gain2/1
  Isq/1 -> Divide/1

== system AM_07_model_pretvornik_FOC/Regulacija2/tokovni_model/Clarke ==
  U_123 : Inport
  ABC_ab1 : Subsystem
  Demux : Demux  Outputs=3
  Mux : Mux  Inputs=2
  U_ab : Outport
  wires:
  U_123/1 -> Demux/1
  Demux/1 -> ABC_ab1/1(A)
  Demux/2 -> ABC_ab1/2(B)
  Demux/3 -> ABC_ab1/3(C)
  ABC_ab1/1(alfa) -> Mux/1
  ABC_ab1/2(beta) -> Mux/2
  Mux/1 -> U_ab/1

== system AM_07_model_pretvornik_FOC/Regulacija2/tokovni_model/Park ==
  U_ab : Inport
  kot : Inport  Port=2
  Demux : Demux  Outputs=2
  Mux : Mux  Inputs=2
  "Sum1 " : Sum  SaturateOnIntegerOverflow=on  InputSameDT=on  OutDataTypeStr=Inherit: Same as first input
  Sum2 : Sum  Inputs=-+  SaturateOnIntegerOverflow=on  InputSameDT=on  OutDataTypeStr=Inherit: Same as first input
  cos : Fcn  Expr=cos(u)
  sin : Fcn  Expr=sin(u)
  x_a*cos : Product  SaturateOnIntegerOverflow=on  RndMeth=Zero  InputSameDT=on  OutDataTypeStr=Inherit: Same as first input
  x_a*sin : Product  SaturateOnIntegerOverflow=on  RndMeth=Zero  InputSameDT=on  OutDataTypeStr=Inherit: Same as first input
  x_b*cos : Product  SaturateOnIntegerOverflow=on  RndMeth=Zero  InputSameDT=on  OutDataTypeStr=Inherit: Same as first input
  "x_b*sin " : Product  SaturateOnIntegerOverflow=on  RndMeth=Zero  InputSameDT=on  OutDataTypeStr=Inherit: Same as first input
  U_dq : Outport
  wires:
  kot/1 -> sin/1, cos/1
  Sum2/1 -> Mux/2
  "Sum1 "/1 -> Mux/1
  x_a*sin/1 -> Sum2/1
  x_b*cos/1 -> Sum2/2
  "x_b*sin "/1 -> "Sum1 "/2
  x_a*cos/1 -> "Sum1 "/1
  sin/1 -> x_a*sin/2, "x_b*sin "/2
  cos/1 -> x_a*cos/2, x_b*cos/2
  Demux/2 -> x_b*cos/1, "x_b*sin "/1
  Demux/1 -> x_a*cos/1, x_a*sin/1
  U_ab/1 -> Demux/1
  Mux/1 -> U_dq/1

== system AM_07_model_pretvornik_FOC/Regulacija2/tokovni_model/eq 5.39 ==
  Isd : Inport
  Discrete-Time Integrator : DiscreteIntegrator  SampleTime=-1  ICPrevOutput=DiscIntNeverNeededParam  ICPrevScaledInput=DiscIntNeverNeededParam
  Gain : Gain  Gain=1/Tr
  Sum : Sum  Inputs=|+-
  Imr : Outport
  dImr/dt : Outport  Port=2
  wires:
  Isd/1 -> Sum/1
  Discrete-Time Integrator/1 -> Imr/1, Sum/2
  Sum/1 -> Gain/1
  Gain/1 -> Discrete-Time Integrator/1, dImr/dt/1

== system AM_07_model_pretvornik_FOC/Regulacija2/tokovni_model/eq 5.40 ==
  Imr : Inport
  Isq : Inport  Port=2
  wr_el : Inport  Port=3
  Add : Sum
  Constant : Constant  Value=0.0001
  Divide : Product  Inputs=*/
  Gain2 : Gain  Gain=Tr
  Sum : Sum  Inputs=|++
  wmr : Outport
  wires:
  Isq/1 -> Divide/1
  Imr/1 -> Gain2/1
  Divide/1 -> Sum/1
  wr_el/1 -> Sum/2
  Sum/1 -> wmr/1
  Gain2/1 -> Add/1
  Add/1 -> Divide/2
  Constant/1 -> Add/2

== system AM_07_model_pretvornik_FOC/ACIM_model/Elektricni del1/Clarke/ABC_ab1 ==
  A : Inport
  B : Inport  Port=2
  C : Inport  Port=3
  Gain1 : Gain  Gain=2
  Gain2 : Gain
  Gain24 : Gain  Gain=sqrt(3)/3
  Sum11 : Sum
  Terminator : Terminator
  alfa : Outport
  beta : Outport  Port=2
  wires:
  A/1 -> Gain2/1, Sum11/1
  Sum11/1 -> Gain24/1
  Gain2/1 -> alfa/1
  Gain24/1 -> beta/1
  B/1 -> Gain1/1
  Gain1/1 -> Sum11/2
  C/1 -> Terminator/1

== system AM_07_model_pretvornik_FOC/ACIM_model/Elektricni del1/Inverzni Clarke/ab_ABC ==
  alfa : Inport
  beta : Inport  Port=2
  Gain1 : Gain
  Gain2 : Gain  Gain=-0.5
  Gain25 : Gain  Gain=sqrt(3)/2
  Gain3 : Gain  Gain=sqrt(3)/2
  Gain4 : Gain  Gain=0.5
  Sum10 : Sum
  Sum11 : Sum  Inputs=--
  A : Outport
  B : Outport  Port=2
  C : Outport  Port=3
  wires:
  Sum11/1 -> C/1
  Sum10/1 -> B/1
  Gain1/1 -> A/1
  alfa/1 -> Gain4/1, Gain2/1, Gain1/1
  Gain2/1 -> Sum10/1
  Gain25/1 -> Sum10/2
  Gain4/1 -> Sum11/1
  beta/1 -> Gain3/1, Gain25/1
  Gain3/1 -> Sum11/2

== system AM_07_model_pretvornik_FOC/ACIM_model/Elektricni del1/napetostni dq model/eq 5.35 ==
  Imr : Inport
  Isq : Inport  Port=2
  Gain : Gain  Gain=3*pp/2
  Gain2 : Gain  Gain=L_m*L_m/L_r
  Product : Product  RndMeth=Zero
  Mel : Outport
  wires:
  Imr/1 -> Product/1
  Isq/1 -> Product/2
  Product/1 -> Gain/1
  Gain2/1 -> Mel/1
  Gain/1 -> Gain2/1

== system AM_07_model_pretvornik_FOC/ACIM_model/Elektricni del1/napetostni dq model/eq 5.39 ==
  Isd : Inport
  Gain : Gain  Gain=1/(L_r/R_r)
  Integrator : Integrator  InitialCondition=1e-3
  Sum : Sum  Inputs=|+-
  Imr : Outport
  dImr/dt : Outport  Port=2
  wires:
  Isd/1 -> Sum/1
  Integrator/1 -> Imr/1, Sum/2
  Sum/1 -> Gain/1
  Gain/1 -> Integrator/1, dImr/dt/1

== system AM_07_model_pretvornik_FOC/ACIM_model/Elektricni del1/napetostni dq model/eq 5.40 ==
  Imr : Inport
  Isq : Inport  Port=2
  wr_el : Inport  Port=3
  Divide : Product  Inputs=*/
  Gain2 : Gain  Gain=(L_r/R_r)
  Saturation : Saturate  UpperLimit=2*pi*500  LowerLimit=-2*pi*500
  Sum : Sum  Inputs=|++
  w_mr : Outport
  wires:
  Isq/1 -> Divide/1
  Imr/1 -> Gain2/1
  Gain2/1 -> Divide/2
  Divide/1 -> Saturation/1  "ws"
  wr_el/1 -> Sum/2
  Sum/1 -> w_mr/1
  Saturation/1 -> Sum/1

== system AM_07_model_pretvornik_FOC/ACIM_model/Elektricni del1/napetostni dq model/eq 5.46 ==
  Usd : Inport
  dImr/dt : Inport  Port=2
  Isq : Inport  Port=3
  wmr : Inport  Port=4
  Gain : Gain  Gain=1/(sigma*L_s)
  Gain1 : Gain  Gain=R_s
  Gain2 : Gain  Gain=(1-sigma)*L_s
  Gain3 : Gain  Gain=sigma*L_s
  Integrator : Integrator
  Product : Product  RndMeth=Zero
  Sum : Sum  Inputs=+--+
  Isd : Outport
  wires:
  Integrator/1 -> Isd/1, Gain1/1
  Gain/1 -> Integrator/1
  Sum/1 -> Gain/1
  Usd/1 -> Sum/1
  Gain1/1 -> Sum/2
  dImr/dt/1 -> Gain2/1
  Gain2/1 -> Sum/3
  wmr/1 -> Product/2
  Isq/1 -> Product/1
  Product/1 -> Gain3/1
  Gain3/1 -> Sum/4

== system AM_07_model_pretvornik_FOC/ACIM_model/Elektricni del1/napetostni dq model/eq 5.47 ==
  Usq : Inport
  Imr : Inport  Port=2
  Isd : Inport  Port=3
  wmr : Inport  Port=4
  Gain : Gain  Gain=1/(sigma*L_s)
  Gain1 : Gain  Gain=R_s
  Gain2 : Gain  Gain=(1-sigma)*L_s
  Gain3 : Gain  Gain=sigma*L_s
  Integrator : Integrator
  Product : Product  RndMeth=Zero
  Product1 : Product  RndMeth=Zero
  Sum : Sum  Inputs=+---
  Isq : Outport
  wires:
  Integrator/1 -> Isq/1, Gain1/1
  Gain/1 -> Integrator/1
  Sum/1 -> Gain/1
  Usq/1 -> Sum/1
  Gain1/1 -> Sum/2
  Imr/1 -> Product/1
  wmr/1 -> Product/2, Product1/1
  Product/1 -> Gain2/1
  Gain2/1 -> Sum/3
  Isd/1 -> Product1/2
  Product1/1 -> Gain3/1
  Gain3/1 -> Sum/4

== system AM_07_model_pretvornik_FOC/ACIM_model1/Elektricni del1/Clarke/ABC_ab1 ==
  A : Inport
  B : Inport  Port=2
  C : Inport  Port=3
  Gain1 : Gain  Gain=2
  Gain2 : Gain
  Gain24 : Gain  Gain=sqrt(3)/3
  Sum11 : Sum
  Terminator : Terminator
  alfa : Outport
  beta : Outport  Port=2
  wires:
  C/1 -> Terminator/1
  Gain1/1 -> Sum11/2
  B/1 -> Gain1/1
  Gain24/1 -> beta/1
  Gain2/1 -> alfa/1
  Sum11/1 -> Gain24/1
  A/1 -> Sum11/1, Gain2/1

== system AM_07_model_pretvornik_FOC/ACIM_model1/Elektricni del1/Inverzni Clarke/ab_ABC ==
  alfa : Inport
  beta : Inport  Port=2
  Gain1 : Gain
  Gain2 : Gain  Gain=-0.5
  Gain25 : Gain  Gain=sqrt(3)/2
  Gain3 : Gain  Gain=sqrt(3)/2
  Gain4 : Gain  Gain=0.5
  Sum10 : Sum
  Sum11 : Sum  Inputs=--
  A : Outport
  B : Outport  Port=2
  C : Outport  Port=3
  wires:
  Gain3/1 -> Sum11/2
  beta/1 -> Gain25/1, Gain3/1
  Gain4/1 -> Sum11/1
  Gain25/1 -> Sum10/2
  Gain2/1 -> Sum10/1
  alfa/1 -> Gain1/1, Gain2/1, Gain4/1
  Gain1/1 -> A/1
  Sum10/1 -> B/1
  Sum11/1 -> C/1

== system AM_07_model_pretvornik_FOC/ACIM_model1/Elektricni del1/napetostni dq model/eq 5.35 ==
  Imr : Inport
  Isq : Inport  Port=2
  Gain : Gain  Gain=3*pp/2
  Gain2 : Gain  Gain=L_m*L_m/L_r
  Product : Product  RndMeth=Zero
  Mel : Outport
  wires:
  Gain/1 -> Gain2/1
  Gain2/1 -> Mel/1
  Product/1 -> Gain/1
  Isq/1 -> Product/2
  Imr/1 -> Product/1

== system AM_07_model_pretvornik_FOC/ACIM_model1/Elektricni del1/napetostni dq model/eq 5.39 ==
  Isd : Inport
  Gain : Gain  Gain=1/(L_r/R_r)
  Integrator : Integrator  InitialCondition=1e-3
  Sum : Sum  Inputs=|+-
  Imr : Outport
  dImr/dt : Outport  Port=2
  wires:
  Gain/1 -> dImr/dt/1, Integrator/1
  Sum/1 -> Gain/1
  Integrator/1 -> Sum/2, Imr/1
  Isd/1 -> Sum/1

== system AM_07_model_pretvornik_FOC/ACIM_model1/Elektricni del1/napetostni dq model/eq 5.40 ==
  Imr : Inport
  Isq : Inport  Port=2
  wr_el : Inport  Port=3
  Divide : Product  Inputs=*/
  Gain2 : Gain  Gain=(L_r/R_r)
  Saturation : Saturate  UpperLimit=2*pi*500  LowerLimit=-2*pi*500
  Sum : Sum  Inputs=|++
  w_mr : Outport
  wires:
  Saturation/1 -> Sum/1
  Sum/1 -> w_mr/1
  wr_el/1 -> Sum/2
  Divide/1 -> Saturation/1  "ws"
  Gain2/1 -> Divide/2
  Imr/1 -> Gain2/1
  Isq/1 -> Divide/1

== system AM_07_model_pretvornik_FOC/ACIM_model1/Elektricni del1/napetostni dq model/eq 5.46 ==
  Usd : Inport
  dImr/dt : Inport  Port=2
  Isq : Inport  Port=3
  wmr : Inport  Port=4
  Gain : Gain  Gain=1/(sigma*L_s)
  Gain1 : Gain  Gain=R_s
  Gain2 : Gain  Gain=(1-sigma)*L_s
  Gain3 : Gain  Gain=sigma*L_s
  Integrator : Integrator
  Product : Product  RndMeth=Zero
  Sum : Sum  Inputs=+--+
  Isd : Outport
  wires:
  Gain3/1 -> Sum/4
  Product/1 -> Gain3/1
  Isq/1 -> Product/1
  wmr/1 -> Product/2
  Gain2/1 -> Sum/3
  dImr/dt/1 -> Gain2/1
  Gain1/1 -> Sum/2
  Usd/1 -> Sum/1
  Sum/1 -> Gain/1
  Gain/1 -> Integrator/1
  Integrator/1 -> Gain1/1, Isd/1

== system AM_07_model_pretvornik_FOC/ACIM_model1/Elektricni del1/napetostni dq model/eq 5.47 ==
  Usq : Inport
  Imr : Inport  Port=2
  Isd : Inport  Port=3
  wmr : Inport  Port=4
  Gain : Gain  Gain=1/(sigma*L_s)
  Gain1 : Gain  Gain=R_s
  Gain2 : Gain  Gain=(1-sigma)*L_s
  Gain3 : Gain  Gain=sigma*L_s
  Integrator : Integrator
  Product : Product  RndMeth=Zero
  Product1 : Product  RndMeth=Zero
  Sum : Sum  Inputs=+---
  Isq : Outport
  wires:
  Gain3/1 -> Sum/4
  Product1/1 -> Gain3/1
  Isd/1 -> Product1/2
  Gain2/1 -> Sum/3
  Product/1 -> Gain2/1
  wmr/1 -> Product1/1, Product/2
  Imr/1 -> Product/1
  Gain1/1 -> Sum/2
  Usq/1 -> Sum/1
  Sum/1 -> Gain/1
  Gain/1 -> Integrator/1
  Integrator/1 -> Gain1/1, Isq/1

== system AM_07_model_pretvornik_FOC/ACIM_model2/Elektricni del1/Clarke/ABC_ab1 ==
  A : Inport
  B : Inport  Port=2
  C : Inport  Port=3
  Gain1 : Gain  Gain=2
  Gain2 : Gain
  Gain24 : Gain  Gain=sqrt(3)/3
  Sum11 : Sum
  Terminator : Terminator
  alfa : Outport
  beta : Outport  Port=2
  wires:
  A/1 -> Gain2/1, Sum11/1
  Sum11/1 -> Gain24/1
  Gain2/1 -> alfa/1
  Gain24/1 -> beta/1
  B/1 -> Gain1/1
  Gain1/1 -> Sum11/2
  C/1 -> Terminator/1

== system AM_07_model_pretvornik_FOC/ACIM_model2/Elektricni del1/Inverzni Clarke/ab_ABC ==
  alfa : Inport
  beta : Inport  Port=2
  Gain1 : Gain
  Gain2 : Gain  Gain=-0.5
  Gain25 : Gain  Gain=sqrt(3)/2
  Gain3 : Gain  Gain=sqrt(3)/2
  Gain4 : Gain  Gain=0.5
  Sum10 : Sum
  Sum11 : Sum  Inputs=--
  A : Outport
  B : Outport  Port=2
  C : Outport  Port=3
  wires:
  Sum11/1 -> C/1
  Sum10/1 -> B/1
  Gain1/1 -> A/1
  alfa/1 -> Gain4/1, Gain2/1, Gain1/1
  Gain2/1 -> Sum10/1
  Gain25/1 -> Sum10/2
  Gain4/1 -> Sum11/1
  beta/1 -> Gain3/1, Gain25/1
  Gain3/1 -> Sum11/2

== system AM_07_model_pretvornik_FOC/ACIM_model2/Elektricni del1/napetostni dq model/eq 5.35 ==
  Imr : Inport
  Isq : Inport  Port=2
  Gain : Gain  Gain=3*pp/2
  Gain2 : Gain  Gain=L_m*L_m/L_r
  Product : Product  RndMeth=Zero
  Mel : Outport
  wires:
  Imr/1 -> Product/1
  Isq/1 -> Product/2
  Product/1 -> Gain/1
  Gain2/1 -> Mel/1
  Gain/1 -> Gain2/1

== system AM_07_model_pretvornik_FOC/ACIM_model2/Elektricni del1/napetostni dq model/eq 5.39 ==
  Isd : Inport
  Gain : Gain  Gain=1/(L_r/R_r)
  Integrator : Integrator  InitialCondition=1e-3
  Sum : Sum  Inputs=|+-
  Imr : Outport
  dImr/dt : Outport  Port=2
  wires:
  Isd/1 -> Sum/1
  Integrator/1 -> Imr/1, Sum/2
  Sum/1 -> Gain/1
  Gain/1 -> Integrator/1, dImr/dt/1

== system AM_07_model_pretvornik_FOC/ACIM_model2/Elektricni del1/napetostni dq model/eq 5.40 ==
  Imr : Inport
  Isq : Inport  Port=2
  wr_el : Inport  Port=3
  Divide : Product  Inputs=*/
  Gain2 : Gain  Gain=(L_r/R_r)
  Saturation : Saturate  UpperLimit=2*pi*500  LowerLimit=-2*pi*500
  Sum : Sum  Inputs=|++
  w_mr : Outport
  wires:
  Isq/1 -> Divide/1
  Imr/1 -> Gain2/1
  Gain2/1 -> Divide/2
  Divide/1 -> Saturation/1  "ws"
  wr_el/1 -> Sum/2
  Sum/1 -> w_mr/1
  Saturation/1 -> Sum/1

== system AM_07_model_pretvornik_FOC/ACIM_model2/Elektricni del1/napetostni dq model/eq 5.46 ==
  Usd : Inport
  dImr/dt : Inport  Port=2
  Isq : Inport  Port=3
  wmr : Inport  Port=4
  Gain : Gain  Gain=1/(sigma*L_s)
  Gain1 : Gain  Gain=R_s
  Gain2 : Gain  Gain=(1-sigma)*L_s
  Gain3 : Gain  Gain=sigma*L_s
  Integrator : Integrator
  Product : Product  RndMeth=Zero
  Sum : Sum  Inputs=+--+
  Isd : Outport
  wires:
  Integrator/1 -> Isd/1, Gain1/1
  Gain/1 -> Integrator/1
  Sum/1 -> Gain/1
  Usd/1 -> Sum/1
  Gain1/1 -> Sum/2
  dImr/dt/1 -> Gain2/1
  Gain2/1 -> Sum/3
  wmr/1 -> Product/2
  Isq/1 -> Product/1
  Product/1 -> Gain3/1
  Gain3/1 -> Sum/4

== system AM_07_model_pretvornik_FOC/ACIM_model2/Elektricni del1/napetostni dq model/eq 5.47 ==
  Usq : Inport
  Imr : Inport  Port=2
  Isd : Inport  Port=3
  wmr : Inport  Port=4
  Gain : Gain  Gain=1/(sigma*L_s)
  Gain1 : Gain  Gain=R_s
  Gain2 : Gain  Gain=(1-sigma)*L_s
  Gain3 : Gain  Gain=sigma*L_s
  Integrator : Integrator
  Product : Product  RndMeth=Zero
  Product1 : Product  RndMeth=Zero
  Sum : Sum  Inputs=+---
  Isq : Outport
  wires:
  Integrator/1 -> Isq/1, Gain1/1
  Gain/1 -> Integrator/1
  Sum/1 -> Gain/1
  Usq/1 -> Sum/1
  Gain1/1 -> Sum/2
  Imr/1 -> Product/1
  wmr/1 -> Product/2, Product1/1
  Product/1 -> Gain2/1
  Gain2/1 -> Sum/3
  Isd/1 -> Product1/2
  Product1/1 -> Gain3/1
  Gain3/1 -> Sum/4

== system AM_07_model_pretvornik_FOC/Regulacija/tokovni_model/Clarke/ABC_ab1 ==
  A : Inport
  B : Inport  Port=2
  C : Inport  Port=3
  Gain1 : Gain  Gain=2
  Gain2 : Gain
  Gain24 : Gain  Gain=sqrt(3)/3
  Sum11 : Sum
  Terminator : Terminator
  alfa : Outport
  beta : Outport  Port=2
  wires:
  A/1 -> Gain2/1, Sum11/1
  Sum11/1 -> Gain24/1
  Gain2/1 -> alfa/1
  Gain24/1 -> beta/1
  B/1 -> Gain1/1
  Gain1/1 -> Sum11/2
  C/1 -> Terminator/1

== system AM_07_model_pretvornik_FOC/Regulacija1/tokovni_model/Clarke/ABC_ab1 ==
  A : Inport
  B : Inport  Port=2
  C : Inport  Port=3
  Gain1 : Gain  Gain=2
  Gain2 : Gain
  Gain24 : Gain  Gain=sqrt(3)/3
  Sum11 : Sum
  Terminator : Terminator
  alfa : Outport
  beta : Outport  Port=2
  wires:
  C/1 -> Terminator/1
  Gain1/1 -> Sum11/2
  B/1 -> Gain1/1
  Gain24/1 -> beta/1
  Gain2/1 -> alfa/1
  Sum11/1 -> Gain24/1
  A/1 -> Sum11/1, Gain2/1

== system AM_07_model_pretvornik_FOC/Regulacija2/tokovni_model/Clarke/ABC_ab1 ==
  A : Inport
  B : Inport  Port=2
  C : Inport  Port=3
  Gain1 : Gain  Gain=2
  Gain2 : Gain
  Gain24 : Gain  Gain=sqrt(3)/3
  Sum11 : Sum
  Terminator : Terminator
  alfa : Outport
  beta : Outport  Port=2
  wires:
  A/1 -> Gain2/1, Sum11/1
  Sum11/1 -> Gain24/1
  Gain2/1 -> alfa/1
  Gain24/1 -> beta/1
  B/1 -> Gain1/1
  Gain1/1 -> Sum11/2
  C/1 -> Terminator/1
